simulink model "P_2_1_h_Kocsi_modell_raketaval"  (R2021b)
settings: Solver=VariableStepAuto  StartTime=0.0  StopTime=40  RelTol=1e-3
settings Model: Creator=davidpaksi  LastModifiedBy=davidpaksi
settings SolverCC: AlgebraicLoopSolver=TrustRegion
settings DebuggingCC: SFMachineParentedDataDiag=warning

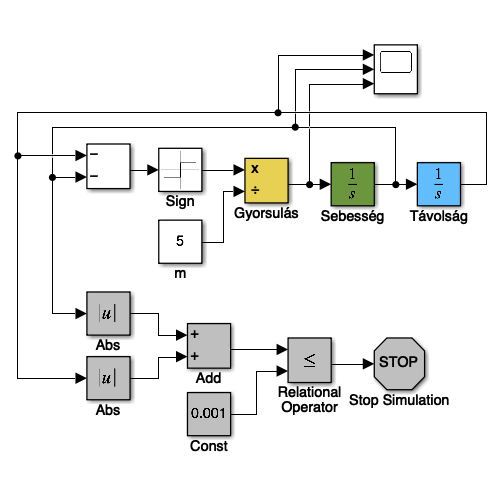
[thumbnail: Simulink's stored preview of the top-level diagram]
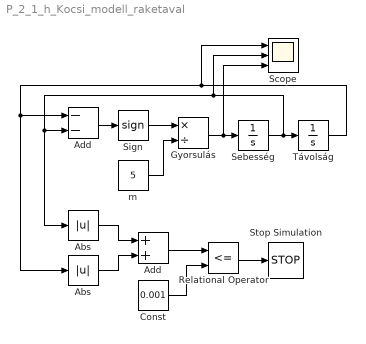
== system P_2_1_h_Kocsi_modell_raketaval ==
  "  Abs  " : Abs
  "  Add  " : Sum
  " Abs " : Abs
  " Gyorsulás " : Product  Inputs=*/
  " Relational Operator " : RelationalOperator  Operator=<=  OutDataTypeStr=boolean  RndMeth=Simplest
  " Sign " : Signum  ZeroCross=off
  " Stop Simulation " : Stop
  Add : Sum  Inputs=--
  Const : Constant  Value=0.001
  Scope : Scope  NumInputPorts=3
  Sebesség : Integrator
  Távolság : Integrator  InitialCondition=5
  m : Constant  Value=5
  wires:
  Const/1 -> " Relational Operator "/2
  " Gyorsulás "/1 -> Scope/3, Sebesség/1
  " Sign "/1 -> " Gyorsulás "/1
  Add/1 -> " Sign "/1
  Távolság/1 -> "  Abs  "/1, Add/1, Scope/1
  " Abs "/1 -> "  Add  "/1
  "  Abs  "/1 -> "  Add  "/2
  "  Add  "/1 -> " Relational Operator "/1
  Sebesség/1 -> " Abs "/1, Add/2, Scope/2, Távolság/1
  " Relational Operator "/1 -> " Stop Simulation "/1
  m/1 -> " Gyorsulás "/2
